simulink model "Malha_aberta_PID_2016"  (R2022b)
settings: Solver=FixedStepAuto  StartTime=0.0  StopTime=250  FixedStep=0.01  RelTol=1e-3
values from neighbouring files (symbols this model uses):
  P_Kp = tal/(K*T)    [Analisa_malha_aberta.m]    (also in Analisa_malha_fechada.m = 0)
  PI_Kp = 0.9*tal/(K*T)    [Analisa_malha_aberta.m]    (also in Analisa_malha_fechada.m = 0)
  PI_Ti = T/0.3    [Analisa_malha_aberta.m]    (also in Analisa_malha_fechada.m = 0)
  PID_Kp = 1.2*tal/(K*T)    [Analisa_malha_aberta.m]    (also in Analisa_malha_fechada.m = 0)
  PID_Td = 0.5*T    [Analisa_malha_aberta.m]    (also in Analisa_malha_fechada.m = 0)
  PID_Ti = 2*T    [Analisa_malha_aberta.m]    (also in Analisa_malha_fechada.m = 0)
settings Model: Creator=Gabriel  LastModifiedBy=mluser
settings SolverCC: AlgebraicLoopSolver=TrustRegion
settings DebuggingCC: ArithmeticOperatorsInVariantConditions=warning
settings ModelReferenceCC: EnableRefExpFcnMdlSchedulingChecks=on
settings SFSimCC: CustomCodeUndefinedFunction=UseInterfaceOnly
settings CodeAppCC: StateflowObjectComments=on

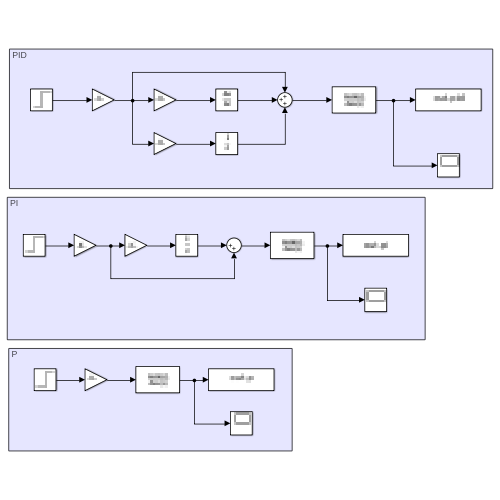
[thumbnail: Simulink's stored preview of the top-level diagram]
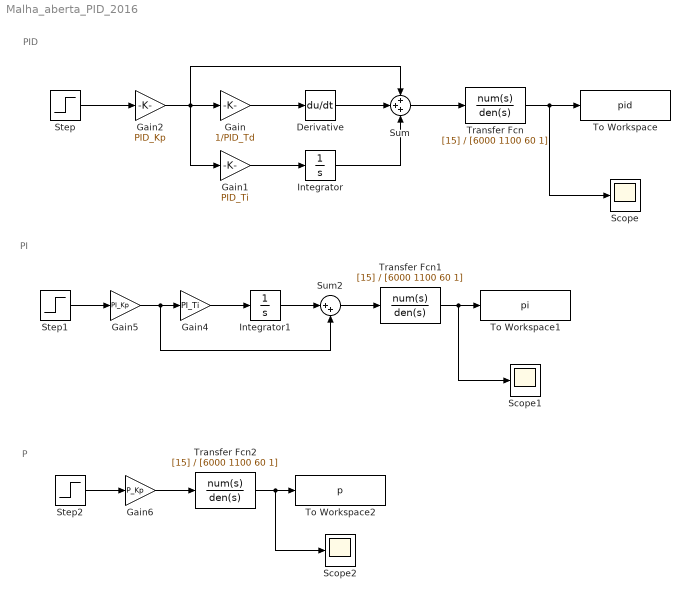
== system Malha_aberta_PID_2016 ==
  note: P
  note: PI
  note: PID
  Derivative : Derivative
  Gain : Gain  Gain=1/PID_Td
  Gain1 : Gain  Gain=PID_Ti
  Gain2 : Gain  Gain=PID_Kp
  Gain4 : Gain  Gain=PI_Ti
  Gain5 : Gain  Gain=PI_Kp
  Gain6 : Gain  Gain=P_Kp
  Integrator : Integrator
  Integrator1 : Integrator
  Scope : Scope
  Scope1 : Scope
  Scope2 : Scope
  Step : Step  SampleTime=0
  Step1 : Step  SampleTime=0
  Step2 : Step  SampleTime=0
  Sum : Sum  Inputs=+++
  Sum2 : Sum  Inputs=|++
  To Workspace : ToWorkspace  VariableName=pid  SampleTime=-1
  To Workspace1 : ToWorkspace  VariableName=pi  SampleTime=-1
  To Workspace2 : ToWorkspace  VariableName=p  SampleTime=-1
  Transfer Fcn : TransferFcn  Numerator=[15]  Denominator=[6000 1100 60 1]
  Transfer Fcn1 : TransferFcn  Numerator=[15]  Denominator=[6000 1100 60 1]
  Transfer Fcn2 : TransferFcn  Numerator=[15]  Denominator=[6000 1100 60 1]
  wires:
  Gain1/1 -> Integrator/1
  Gain/1 -> Derivative/1
  Derivative/1 -> Sum/2
  Integrator/1 -> Sum/3
  Gain2/1 -> Gain1/1, Gain/1, Sum/1
  Sum/1 -> Transfer Fcn/1
  Transfer Fcn/1 -> Scope/1, To Workspace/1
  Transfer Fcn1/1 -> To Workspace1/1, Scope1/1
  Sum2/1 -> Transfer Fcn1/1
  Gain4/1 -> Integrator1/1
  Gain5/1 -> Sum2/2, Gain4/1
  Integrator1/1 -> Sum2/1
  Transfer Fcn2/1 -> To Workspace2/1, Scope2/1
  Gain6/1 -> Transfer Fcn2/1
  Step/1 -> Gain2/1
  Step1/1 -> Gain5/1
  Step2/1 -> Gain6/1
